simulink model "rx2"  (R2022b)
settings: Solver=FixedStepDiscrete  StartTime=0.0  StopTime=3.3E6  FixedStep=1  RelTol=1e-3  EnableMultiTasking=on
model workspace (MAT data in the model file):
  mwTaskManagerKernelLatency = 0
undefined symbols (not defined in the file or in its folder): Add, jsin, magnitude, rom_pilot_conj_tt, Shift
libraries: hdlsllib x3231, whdlutilities x525, simulink x260, whdlmod x112, whdledac x26, dsphdlmathfun2 x24, commchan3 x1
(part 59 of 59)

== system rx2/process8/decoder/p-p/Subsystem2/Subsystem1/Subsystem1/Subsystem/Subsystem1/Subsystem1 ==
  data : Inport  OutDataTypeStr=data_type
  wr_addr : Inport  Port=2
  wr_en : Inport  Port=3
  rd_addr : Inport  Port=4
  Demux : Demux  Outputs=2
  Mux : Mux  Inputs=2
  Simple Dual Port RAM : hdlsllib/HDL RAMs/Simple Dual Port RAM  ram_size=address_len
  Simple Dual Port RAM1 : hdlsllib/HDL RAMs/Simple Dual Port RAM  ram_size=address_len
  rd_dout : Outport  PortDimensions=2  VectorParamsAs1DForOutWhenUnconnected=off
  wires:
  Mux/1 -> rd_dout/1
  Simple Dual Port RAM/1 -> Mux/1
  Simple Dual Port RAM1/1 -> Mux/2
  data/1 -> Demux/1
  Demux/1 -> Simple Dual Port RAM/1
  Demux/2 -> Simple Dual Port RAM1/1
  wr_addr/1 -> Simple Dual Port RAM1/2, Simple Dual Port RAM/2
  wr_en/1 -> Simple Dual Port RAM/3, Simple Dual Port RAM1/3
  rd_addr/1 -> Simple Dual Port RAM/4, Simple Dual Port RAM1/4

== system rx2/process8/decoder/p-p/Subsystem2/Subsystem1/Subsystem1/Subsystem/Subsystem4/Subsystem ==
  data : Inport  OutDataTypeStr=data_type
  wr_addr : Inport  Port=2
  wr_en : Inport  Port=3
  rd_addr : Inport  Port=4
  Demux : Demux  Outputs=2
  Mux : Mux  Inputs=2
  Simple Dual Port RAM : hdlsllib/HDL RAMs/Simple Dual Port RAM  ram_size=address_len
  Simple Dual Port RAM1 : hdlsllib/HDL RAMs/Simple Dual Port RAM  ram_size=address_len
  rd_dout : Outport  PortDimensions=2  VectorParamsAs1DForOutWhenUnconnected=off
  wires:
  Mux/1 -> rd_dout/1
  Simple Dual Port RAM/1 -> Mux/1
  Simple Dual Port RAM1/1 -> Mux/2
  data/1 -> Demux/1
  Demux/1 -> Simple Dual Port RAM/1
  Demux/2 -> Simple Dual Port RAM1/1
  wr_addr/1 -> Simple Dual Port RAM1/2, Simple Dual Port RAM/2
  wr_en/1 -> Simple Dual Port RAM/3, Simple Dual Port RAM1/3
  rd_addr/1 -> Simple Dual Port RAM/4, Simple Dual Port RAM1/4

== system rx2/process8/decoder/p-p/Subsystem2/Subsystem1/Subsystem1/Subsystem/Subsystem4/Subsystem1 ==
  data : Inport  OutDataTypeStr=data_type
  wr_addr : Inport  Port=2
  wr_en : Inport  Port=3
  rd_addr : Inport  Port=4
  Demux : Demux  Outputs=2
  Mux : Mux  Inputs=2
  Simple Dual Port RAM : hdlsllib/HDL RAMs/Simple Dual Port RAM  ram_size=address_len
  Simple Dual Port RAM1 : hdlsllib/HDL RAMs/Simple Dual Port RAM  ram_size=address_len
  rd_dout : Outport  PortDimensions=2  VectorParamsAs1DForOutWhenUnconnected=off
  wires:
  rd_addr/1 -> Simple Dual Port RAM1/4, Simple Dual Port RAM/4
  wr_en/1 -> Simple Dual Port RAM1/3, Simple Dual Port RAM/3
  wr_addr/1 -> Simple Dual Port RAM/2, Simple Dual Port RAM1/2
  Demux/2 -> Simple Dual Port RAM1/1
  Demux/1 -> Simple Dual Port RAM/1
  data/1 -> Demux/1
  Simple Dual Port RAM1/1 -> Mux/2
  Simple Dual Port RAM/1 -> Mux/1
  Mux/1 -> rd_dout/1

== system rx2/process8/decoder/p-p/Subsystem2/Subsystem1/Subsystem1/Subsystem1/Subsystem1/Subsystem ==
  data : Inport  OutDataTypeStr=data_type
  wr_addr : Inport  Port=2
  wr_en : Inport  Port=3
  rd_addr : Inport  Port=4
  Demux : Demux  Outputs=2
  Mux : Mux  Inputs=2
  Simple Dual Port RAM : hdlsllib/HDL RAMs/Simple Dual Port RAM  ram_size=address_len
  Simple Dual Port RAM1 : hdlsllib/HDL RAMs/Simple Dual Port RAM  ram_size=address_len
  rd_dout : Outport  PortDimensions=2  VectorParamsAs1DForOutWhenUnconnected=off
  wires:
  rd_addr/1 -> Simple Dual Port RAM1/4, Simple Dual Port RAM/4
  wr_en/1 -> Simple Dual Port RAM1/3, Simple Dual Port RAM/3
  wr_addr/1 -> Simple Dual Port RAM/2, Simple Dual Port RAM1/2
  Demux/2 -> Simple Dual Port RAM1/1
  Demux/1 -> Simple Dual Port RAM/1
  data/1 -> Demux/1
  Simple Dual Port RAM1/1 -> Mux/2
  Simple Dual Port RAM/1 -> Mux/1
  Mux/1 -> rd_dout/1

== system rx2/process8/decoder/p-p/Subsystem2/Subsystem1/Subsystem1/Subsystem1/Subsystem1/Subsystem1 ==
  data : Inport  OutDataTypeStr=data_type
  wr_addr : Inport  Port=2
  wr_en : Inport  Port=3
  rd_addr : Inport  Port=4
  Demux : Demux  Outputs=2
  Mux : Mux  Inputs=2
  Simple Dual Port RAM : hdlsllib/HDL RAMs/Simple Dual Port RAM  ram_size=address_len
  Simple Dual Port RAM1 : hdlsllib/HDL RAMs/Simple Dual Port RAM  ram_size=address_len
  rd_dout : Outport  PortDimensions=2  VectorParamsAs1DForOutWhenUnconnected=off
  wires:
  Mux/1 -> rd_dout/1
  Simple Dual Port RAM/1 -> Mux/1
  Simple Dual Port RAM1/1 -> Mux/2
  data/1 -> Demux/1
  Demux/1 -> Simple Dual Port RAM/1
  Demux/2 -> Simple Dual Port RAM1/1
  wr_addr/1 -> Simple Dual Port RAM1/2, Simple Dual Port RAM/2
  wr_en/1 -> Simple Dual Port RAM/3, Simple Dual Port RAM1/3
  rd_addr/1 -> Simple Dual Port RAM/4, Simple Dual Port RAM1/4

== system rx2/process8/decoder/p-p/Subsystem2/Subsystem1/Subsystem1/Subsystem1/Subsystem4/Subsystem ==
  data : Inport  OutDataTypeStr=data_type
  wr_addr : Inport  Port=2
  wr_en : Inport  Port=3
  rd_addr : Inport  Port=4
  Demux : Demux  Outputs=2
  Mux : Mux  Inputs=2
  Simple Dual Port RAM : hdlsllib/HDL RAMs/Simple Dual Port RAM  ram_size=address_len
  Simple Dual Port RAM1 : hdlsllib/HDL RAMs/Simple Dual Port RAM  ram_size=address_len
  rd_dout : Outport  PortDimensions=2  VectorParamsAs1DForOutWhenUnconnected=off
  wires:
  rd_addr/1 -> Simple Dual Port RAM1/4, Simple Dual Port RAM/4
  wr_en/1 -> Simple Dual Port RAM1/3, Simple Dual Port RAM/3
  wr_addr/1 -> Simple Dual Port RAM/2, Simple Dual Port RAM1/2
  Demux/2 -> Simple Dual Port RAM1/1
  Demux/1 -> Simple Dual Port RAM/1
  data/1 -> Demux/1
  Simple Dual Port RAM1/1 -> Mux/2
  Simple Dual Port RAM/1 -> Mux/1
  Mux/1 -> rd_dout/1

== system rx2/process8/decoder/p-p/Subsystem2/Subsystem1/Subsystem1/Subsystem1/Subsystem4/Subsystem1 ==
  data : Inport  OutDataTypeStr=data_type
  wr_addr : Inport  Port=2
  wr_en : Inport  Port=3
  rd_addr : Inport  Port=4
  Demux : Demux  Outputs=2
  Mux : Mux  Inputs=2
  Simple Dual Port RAM : hdlsllib/HDL RAMs/Simple Dual Port RAM  ram_size=address_len
  Simple Dual Port RAM1 : hdlsllib/HDL RAMs/Simple Dual Port RAM  ram_size=address_len
  rd_dout : Outport  PortDimensions=2  VectorParamsAs1DForOutWhenUnconnected=off
  wires:
  Mux/1 -> rd_dout/1
  Simple Dual Port RAM/1 -> Mux/1
  Simple Dual Port RAM1/1 -> Mux/2
  data/1 -> Demux/1
  Demux/1 -> Simple Dual Port RAM/1
  Demux/2 -> Simple Dual Port RAM1/1
  wr_addr/1 -> Simple Dual Port RAM1/2, Simple Dual Port RAM/2
  wr_en/1 -> Simple Dual Port RAM/3, Simple Dual Port RAM1/3
  rd_addr/1 -> Simple Dual Port RAM/4, Simple Dual Port RAM1/4

== system rx2/process8/decoder/p-p/Subsystem2/Subsystem1/Subsystem2/Subsystem/Subsystem1/Subsystem ==
  data : Inport  OutDataTypeStr=data_type
  wr_addr : Inport  Port=2
  wr_en : Inport  Port=3
  rd_addr : Inport  Port=4
  Demux : Demux  Outputs=2
  Mux : Mux  Inputs=2
  Simple Dual Port RAM : hdlsllib/HDL RAMs/Simple Dual Port RAM  ram_size=address_len
  Simple Dual Port RAM1 : hdlsllib/HDL RAMs/Simple Dual Port RAM  ram_size=address_len
  rd_dout : Outport  PortDimensions=2  VectorParamsAs1DForOutWhenUnconnected=off
  wires:
  rd_addr/1 -> Simple Dual Port RAM1/4, Simple Dual Port RAM/4
  wr_en/1 -> Simple Dual Port RAM1/3, Simple Dual Port RAM/3
  wr_addr/1 -> Simple Dual Port RAM/2, Simple Dual Port RAM1/2
  Demux/2 -> Simple Dual Port RAM1/1
  Demux/1 -> Simple Dual Port RAM/1
  data/1 -> Demux/1
  Simple Dual Port RAM1/1 -> Mux/2
  Simple Dual Port RAM/1 -> Mux/1
  Mux/1 -> rd_dout/1

== system rx2/process8/decoder/p-p/Subsystem2/Subsystem1/Subsystem2/Subsystem/Subsystem1/Subsystem1 ==
  data : Inport  OutDataTypeStr=data_type
  wr_addr : Inport  Port=2
  wr_en : Inport  Port=3
  rd_addr : Inport  Port=4
  Demux : Demux  Outputs=2
  Mux : Mux  Inputs=2
  Simple Dual Port RAM : hdlsllib/HDL RAMs/Simple Dual Port RAM  ram_size=address_len
  Simple Dual Port RAM1 : hdlsllib/HDL RAMs/Simple Dual Port RAM  ram_size=address_len
  rd_dout : Outport  PortDimensions=2  VectorParamsAs1DForOutWhenUnconnected=off
  wires:
  Mux/1 -> rd_dout/1
  Simple Dual Port RAM/1 -> Mux/1
  Simple Dual Port RAM1/1 -> Mux/2
  data/1 -> Demux/1
  Demux/1 -> Simple Dual Port RAM/1
  Demux/2 -> Simple Dual Port RAM1/1
  wr_addr/1 -> Simple Dual Port RAM1/2, Simple Dual Port RAM/2
  wr_en/1 -> Simple Dual Port RAM/3, Simple Dual Port RAM1/3
  rd_addr/1 -> Simple Dual Port RAM/4, Simple Dual Port RAM1/4

== system rx2/process8/decoder/p-p/Subsystem2/Subsystem1/Subsystem2/Subsystem/Subsystem4/Subsystem ==
  data : Inport  OutDataTypeStr=data_type
  wr_addr : Inport  Port=2
  wr_en : Inport  Port=3
  rd_addr : Inport  Port=4
  Demux : Demux  Outputs=2
  Mux : Mux  Inputs=2
  Simple Dual Port RAM : hdlsllib/HDL RAMs/Simple Dual Port RAM  ram_size=address_len
  Simple Dual Port RAM1 : hdlsllib/HDL RAMs/Simple Dual Port RAM  ram_size=address_len
  rd_dout : Outport  PortDimensions=2  VectorParamsAs1DForOutWhenUnconnected=off
  wires:
  Mux/1 -> rd_dout/1
  Simple Dual Port RAM/1 -> Mux/1
  Simple Dual Port RAM1/1 -> Mux/2
  data/1 -> Demux/1
  Demux/1 -> Simple Dual Port RAM/1
  Demux/2 -> Simple Dual Port RAM1/1
  wr_addr/1 -> Simple Dual Port RAM1/2, Simple Dual Port RAM/2
  wr_en/1 -> Simple Dual Port RAM/3, Simple Dual Port RAM1/3
  rd_addr/1 -> Simple Dual Port RAM/4, Simple Dual Port RAM1/4

== system rx2/process8/decoder/p-p/Subsystem2/Subsystem1/Subsystem2/Subsystem/Subsystem4/Subsystem1 ==
  data : Inport  OutDataTypeStr=data_type
  wr_addr : Inport  Port=2
  wr_en : Inport  Port=3
  rd_addr : Inport  Port=4
  Demux : Demux  Outputs=2
  Mux : Mux  Inputs=2
  Simple Dual Port RAM : hdlsllib/HDL RAMs/Simple Dual Port RAM  ram_size=address_len
  Simple Dual Port RAM1 : hdlsllib/HDL RAMs/Simple Dual Port RAM  ram_size=address_len
  rd_dout : Outport  PortDimensions=2  VectorParamsAs1DForOutWhenUnconnected=off
  wires:
  rd_addr/1 -> Simple Dual Port RAM1/4, Simple Dual Port RAM/4
  wr_en/1 -> Simple Dual Port RAM1/3, Simple Dual Port RAM/3
  wr_addr/1 -> Simple Dual Port RAM/2, Simple Dual Port RAM1/2
  Demux/2 -> Simple Dual Port RAM1/1
  Demux/1 -> Simple Dual Port RAM/1
  data/1 -> Demux/1
  Simple Dual Port RAM1/1 -> Mux/2
  Simple Dual Port RAM/1 -> Mux/1
  Mux/1 -> rd_dout/1

== system rx2/process8/decoder/p-p/Subsystem2/Subsystem1/Subsystem2/Subsystem1/Subsystem1/Subsystem ==
  data : Inport  OutDataTypeStr=data_type
  wr_addr : Inport  Port=2
  wr_en : Inport  Port=3
  rd_addr : Inport  Port=4
  Demux : Demux  Outputs=2
  Mux : Mux  Inputs=2
  Simple Dual Port RAM : hdlsllib/HDL RAMs/Simple Dual Port RAM  ram_size=address_len
  Simple Dual Port RAM1 : hdlsllib/HDL RAMs/Simple Dual Port RAM  ram_size=address_len
  rd_dout : Outport  PortDimensions=2  VectorParamsAs1DForOutWhenUnconnected=off
  wires:
  rd_addr/1 -> Simple Dual Port RAM1/4, Simple Dual Port RAM/4
  wr_en/1 -> Simple Dual Port RAM1/3, Simple Dual Port RAM/3
  wr_addr/1 -> Simple Dual Port RAM/2, Simple Dual Port RAM1/2
  Demux/2 -> Simple Dual Port RAM1/1
  Demux/1 -> Simple Dual Port RAM/1
  data/1 -> Demux/1
  Simple Dual Port RAM1/1 -> Mux/2
  Simple Dual Port RAM/1 -> Mux/1
  Mux/1 -> rd_dout/1

== system rx2/process8/decoder/p-p/Subsystem2/Subsystem1/Subsystem2/Subsystem1/Subsystem1/Subsystem1 ==
  data : Inport  OutDataTypeStr=data_type
  wr_addr : Inport  Port=2
  wr_en : Inport  Port=3
  rd_addr : Inport  Port=4
  Demux : Demux  Outputs=2
  Mux : Mux  Inputs=2
  Simple Dual Port RAM : hdlsllib/HDL RAMs/Simple Dual Port RAM  ram_size=address_len
  Simple Dual Port RAM1 : hdlsllib/HDL RAMs/Simple Dual Port RAM  ram_size=address_len
  rd_dout : Outport  PortDimensions=2  VectorParamsAs1DForOutWhenUnconnected=off
  wires:
  Mux/1 -> rd_dout/1
  Simple Dual Port RAM/1 -> Mux/1
  Simple Dual Port RAM1/1 -> Mux/2
  data/1 -> Demux/1
  Demux/1 -> Simple Dual Port RAM/1
  Demux/2 -> Simple Dual Port RAM1/1
  wr_addr/1 -> Simple Dual Port RAM1/2, Simple Dual Port RAM/2
  wr_en/1 -> Simple Dual Port RAM/3, Simple Dual Port RAM1/3
  rd_addr/1 -> Simple Dual Port RAM/4, Simple Dual Port RAM1/4

== system rx2/process8/decoder/p-p/Subsystem2/Subsystem1/Subsystem2/Subsystem1/Subsystem4/Subsystem ==
  data : Inport  OutDataTypeStr=data_type
  wr_addr : Inport  Port=2
  wr_en : Inport  Port=3
  rd_addr : Inport  Port=4
  Demux : Demux  Outputs=2
  Mux : Mux  Inputs=2
  Simple Dual Port RAM : hdlsllib/HDL RAMs/Simple Dual Port RAM  ram_size=address_len
  Simple Dual Port RAM1 : hdlsllib/HDL RAMs/Simple Dual Port RAM  ram_size=address_len
  rd_dout : Outport  PortDimensions=2  VectorParamsAs1DForOutWhenUnconnected=off
  wires:
  rd_addr/1 -> Simple Dual Port RAM1/4, Simple Dual Port RAM/4
  wr_en/1 -> Simple Dual Port RAM1/3, Simple Dual Port RAM/3
  wr_addr/1 -> Simple Dual Port RAM/2, Simple Dual Port RAM1/2
  Demux/2 -> Simple Dual Port RAM1/1
  Demux/1 -> Simple Dual Port RAM/1
  data/1 -> Demux/1
  Simple Dual Port RAM1/1 -> Mux/2
  Simple Dual Port RAM/1 -> Mux/1
  Mux/1 -> rd_dout/1

== system rx2/process8/decoder/p-p/Subsystem2/Subsystem1/Subsystem2/Subsystem1/Subsystem4/Subsystem1 ==
  data : Inport  OutDataTypeStr=data_type
  wr_addr : Inport  Port=2
  wr_en : Inport  Port=3
  rd_addr : Inport  Port=4
  Demux : Demux  Outputs=2
  Mux : Mux  Inputs=2
  Simple Dual Port RAM : hdlsllib/HDL RAMs/Simple Dual Port RAM  ram_size=address_len
  Simple Dual Port RAM1 : hdlsllib/HDL RAMs/Simple Dual Port RAM  ram_size=address_len
  rd_dout : Outport  PortDimensions=2  VectorParamsAs1DForOutWhenUnconnected=off
  wires:
  Mux/1 -> rd_dout/1
  Simple Dual Port RAM/1 -> Mux/1
  Simple Dual Port RAM1/1 -> Mux/2
  data/1 -> Demux/1
  Demux/1 -> Simple Dual Port RAM/1
  Demux/2 -> Simple Dual Port RAM1/1
  wr_addr/1 -> Simple Dual Port RAM1/2, Simple Dual Port RAM/2
  wr_en/1 -> Simple Dual Port RAM/3, Simple Dual Port RAM1/3
  rd_addr/1 -> Simple Dual Port RAM/4, Simple Dual Port RAM1/4

== system rx2/process9/decoder/p-p/Subsystem2/Subsystem/Subsystem1/Subsystem/Subsystem1/Subsystem ==
  data : Inport  OutDataTypeStr=data_type
  wr_addr : Inport  Port=2
  wr_en : Inport  Port=3
  rd_addr : Inport  Port=4
  Demux : Demux  Outputs=2
  Mux : Mux  Inputs=2
  Simple Dual Port RAM : hdlsllib/HDL RAMs/Simple Dual Port RAM  ram_size=address_len
  Simple Dual Port RAM1 : hdlsllib/HDL RAMs/Simple Dual Port RAM  ram_size=address_len
  rd_dout : Outport  PortDimensions=2  VectorParamsAs1DForOutWhenUnconnected=off
  wires:
  Mux/1 -> rd_dout/1
  Simple Dual Port RAM/1 -> Mux/1
  Simple Dual Port RAM1/1 -> Mux/2
  data/1 -> Demux/1
  Demux/1 -> Simple Dual Port RAM/1
  Demux/2 -> Simple Dual Port RAM1/1
  wr_addr/1 -> Simple Dual Port RAM1/2, Simple Dual Port RAM/2
  wr_en/1 -> Simple Dual Port RAM/3, Simple Dual Port RAM1/3
  rd_addr/1 -> Simple Dual Port RAM/4, Simple Dual Port RAM1/4

== system rx2/process9/decoder/p-p/Subsystem2/Subsystem/Subsystem1/Subsystem/Subsystem1/Subsystem1 ==
  data : Inport  OutDataTypeStr=data_type
  wr_addr : Inport  Port=2
  wr_en : Inport  Port=3
  rd_addr : Inport  Port=4
  Demux : Demux  Outputs=2
  Mux : Mux  Inputs=2
  Simple Dual Port RAM : hdlsllib/HDL RAMs/Simple Dual Port RAM  ram_size=address_len
  Simple Dual Port RAM1 : hdlsllib/HDL RAMs/Simple Dual Port RAM  ram_size=address_len
  rd_dout : Outport  PortDimensions=2  VectorParamsAs1DForOutWhenUnconnected=off
  wires:
  rd_addr/1 -> Simple Dual Port RAM1/4, Simple Dual Port RAM/4
  wr_en/1 -> Simple Dual Port RAM1/3, Simple Dual Port RAM/3
  wr_addr/1 -> Simple Dual Port RAM/2, Simple Dual Port RAM1/2
  Demux/2 -> Simple Dual Port RAM1/1
  Demux/1 -> Simple Dual Port RAM/1
  data/1 -> Demux/1
  Simple Dual Port RAM1/1 -> Mux/2
  Simple Dual Port RAM/1 -> Mux/1
  Mux/1 -> rd_dout/1

== system rx2/process9/decoder/p-p/Subsystem2/Subsystem/Subsystem1/Subsystem/Subsystem4/Subsystem ==
  data : Inport  OutDataTypeStr=data_type
  wr_addr : Inport  Port=2
  wr_en : Inport  Port=3
  rd_addr : Inport  Port=4
  Demux : Demux  Outputs=2
  Mux : Mux  Inputs=2
  Simple Dual Port RAM : hdlsllib/HDL RAMs/Simple Dual Port RAM  ram_size=address_len
  Simple Dual Port RAM1 : hdlsllib/HDL RAMs/Simple Dual Port RAM  ram_size=address_len
  rd_dout : Outport  PortDimensions=2  VectorParamsAs1DForOutWhenUnconnected=off
  wires:
  rd_addr/1 -> Simple Dual Port RAM1/4, Simple Dual Port RAM/4
  wr_en/1 -> Simple Dual Port RAM1/3, Simple Dual Port RAM/3
  wr_addr/1 -> Simple Dual Port RAM/2, Simple Dual Port RAM1/2
  Demux/2 -> Simple Dual Port RAM1/1
  Demux/1 -> Simple Dual Port RAM/1
  data/1 -> Demux/1
  Simple Dual Port RAM1/1 -> Mux/2
  Simple Dual Port RAM/1 -> Mux/1
  Mux/1 -> rd_dout/1

== system rx2/process9/decoder/p-p/Subsystem2/Subsystem/Subsystem1/Subsystem/Subsystem4/Subsystem1 ==
  data : Inport  OutDataTypeStr=data_type
  wr_addr : Inport  Port=2
  wr_en : Inport  Port=3
  rd_addr : Inport  Port=4
  Demux : Demux  Outputs=2
  Mux : Mux  Inputs=2
  Simple Dual Port RAM : hdlsllib/HDL RAMs/Simple Dual Port RAM  ram_size=address_len
  Simple Dual Port RAM1 : hdlsllib/HDL RAMs/Simple Dual Port RAM  ram_size=address_len
  rd_dout : Outport  PortDimensions=2  VectorParamsAs1DForOutWhenUnconnected=off
  wires:
  Mux/1 -> rd_dout/1
  Simple Dual Port RAM/1 -> Mux/1
  Simple Dual Port RAM1/1 -> Mux/2
  data/1 -> Demux/1
  Demux/1 -> Simple Dual Port RAM/1
  Demux/2 -> Simple Dual Port RAM1/1
  wr_addr/1 -> Simple Dual Port RAM1/2, Simple Dual Port RAM/2
  wr_en/1 -> Simple Dual Port RAM/3, Simple Dual Port RAM1/3
  rd_addr/1 -> Simple Dual Port RAM/4, Simple Dual Port RAM1/4

== system rx2/process9/decoder/p-p/Subsystem2/Subsystem/Subsystem1/Subsystem1/Subsystem1/Subsystem ==
  data : Inport  OutDataTypeStr=data_type
  wr_addr : Inport  Port=2
  wr_en : Inport  Port=3
  rd_addr : Inport  Port=4
  Demux : Demux  Outputs=2
  Mux : Mux  Inputs=2
  Simple Dual Port RAM : hdlsllib/HDL RAMs/Simple Dual Port RAM  ram_size=address_len
  Simple Dual Port RAM1 : hdlsllib/HDL RAMs/Simple Dual Port RAM  ram_size=address_len
  rd_dout : Outport  PortDimensions=2  VectorParamsAs1DForOutWhenUnconnected=off
  wires:
  Mux/1 -> rd_dout/1
  Simple Dual Port RAM/1 -> Mux/1
  Simple Dual Port RAM1/1 -> Mux/2
  data/1 -> Demux/1
  Demux/1 -> Simple Dual Port RAM/1
  Demux/2 -> Simple Dual Port RAM1/1
  wr_addr/1 -> Simple Dual Port RAM1/2, Simple Dual Port RAM/2
  wr_en/1 -> Simple Dual Port RAM/3, Simple Dual Port RAM1/3
  rd_addr/1 -> Simple Dual Port RAM/4, Simple Dual Port RAM1/4

== system rx2/process9/decoder/p-p/Subsystem2/Subsystem/Subsystem1/Subsystem1/Subsystem1/Subsystem1 ==
  data : Inport  OutDataTypeStr=data_type
  wr_addr : Inport  Port=2
  wr_en : Inport  Port=3
  rd_addr : Inport  Port=4
  Demux : Demux  Outputs=2
  Mux : Mux  Inputs=2
  Simple Dual Port RAM : hdlsllib/HDL RAMs/Simple Dual Port RAM  ram_size=address_len
  Simple Dual Port RAM1 : hdlsllib/HDL RAMs/Simple Dual Port RAM  ram_size=address_len
  rd_dout : Outport  PortDimensions=2  VectorParamsAs1DForOutWhenUnconnected=off
  wires:
  rd_addr/1 -> Simple Dual Port RAM1/4, Simple Dual Port RAM/4
  wr_en/1 -> Simple Dual Port RAM1/3, Simple Dual Port RAM/3
  wr_addr/1 -> Simple Dual Port RAM/2, Simple Dual Port RAM1/2
  Demux/2 -> Simple Dual Port RAM1/1
  Demux/1 -> Simple Dual Port RAM/1
  data/1 -> Demux/1
  Simple Dual Port RAM1/1 -> Mux/2
  Simple Dual Port RAM/1 -> Mux/1
  Mux/1 -> rd_dout/1

== system rx2/process9/decoder/p-p/Subsystem2/Subsystem/Subsystem1/Subsystem1/Subsystem4/Subsystem ==
  data : Inport  OutDataTypeStr=data_type
  wr_addr : Inport  Port=2
  wr_en : Inport  Port=3
  rd_addr : Inport  Port=4
  Demux : Demux  Outputs=2
  Mux : Mux  Inputs=2
  Simple Dual Port RAM : hdlsllib/HDL RAMs/Simple Dual Port RAM  ram_size=address_len
  Simple Dual Port RAM1 : hdlsllib/HDL RAMs/Simple Dual Port RAM  ram_size=address_len
  rd_dout : Outport  PortDimensions=2  VectorParamsAs1DForOutWhenUnconnected=off
  wires:
  Mux/1 -> rd_dout/1
  Simple Dual Port RAM/1 -> Mux/1
  Simple Dual Port RAM1/1 -> Mux/2
  data/1 -> Demux/1
  Demux/1 -> Simple Dual Port RAM/1
  Demux/2 -> Simple Dual Port RAM1/1
  wr_addr/1 -> Simple Dual Port RAM1/2, Simple Dual Port RAM/2
  wr_en/1 -> Simple Dual Port RAM/3, Simple Dual Port RAM1/3
  rd_addr/1 -> Simple Dual Port RAM/4, Simple Dual Port RAM1/4

== system rx2/process9/decoder/p-p/Subsystem2/Subsystem/Subsystem1/Subsystem1/Subsystem4/Subsystem1 ==
  data : Inport  OutDataTypeStr=data_type
  wr_addr : Inport  Port=2
  wr_en : Inport  Port=3
  rd_addr : Inport  Port=4
  Demux : Demux  Outputs=2
  Mux : Mux  Inputs=2
  Simple Dual Port RAM : hdlsllib/HDL RAMs/Simple Dual Port RAM  ram_size=address_len
  Simple Dual Port RAM1 : hdlsllib/HDL RAMs/Simple Dual Port RAM  ram_size=address_len
  rd_dout : Outport  PortDimensions=2  VectorParamsAs1DForOutWhenUnconnected=off
  wires:
  rd_addr/1 -> Simple Dual Port RAM1/4, Simple Dual Port RAM/4
  wr_en/1 -> Simple Dual Port RAM1/3, Simple Dual Port RAM/3
  wr_addr/1 -> Simple Dual Port RAM/2, Simple Dual Port RAM1/2
  Demux/2 -> Simple Dual Port RAM1/1
  Demux/1 -> Simple Dual Port RAM/1
  data/1 -> Demux/1
  Simple Dual Port RAM1/1 -> Mux/2
  Simple Dual Port RAM/1 -> Mux/1
  Mux/1 -> rd_dout/1

== system rx2/process9/decoder/p-p/Subsystem2/Subsystem/Subsystem2/Subsystem/Subsystem1/Subsystem ==
  data : Inport  OutDataTypeStr=data_type
  wr_addr : Inport  Port=2
  wr_en : Inport  Port=3
  rd_addr : Inport  Port=4
  Demux : Demux  Outputs=2
  Mux : Mux  Inputs=2
  Simple Dual Port RAM : hdlsllib/HDL RAMs/Simple Dual Port RAM  ram_size=address_len
  Simple Dual Port RAM1 : hdlsllib/HDL RAMs/Simple Dual Port RAM  ram_size=address_len
  rd_dout : Outport  PortDimensions=2  VectorParamsAs1DForOutWhenUnconnected=off
  wires:
  Mux/1 -> rd_dout/1
  Simple Dual Port RAM/1 -> Mux/1
  Simple Dual Port RAM1/1 -> Mux/2
  data/1 -> Demux/1
  Demux/1 -> Simple Dual Port RAM/1
  Demux/2 -> Simple Dual Port RAM1/1
  wr_addr/1 -> Simple Dual Port RAM1/2, Simple Dual Port RAM/2
  wr_en/1 -> Simple Dual Port RAM/3, Simple Dual Port RAM1/3
  rd_addr/1 -> Simple Dual Port RAM/4, Simple Dual Port RAM1/4

== system rx2/process9/decoder/p-p/Subsystem2/Subsystem/Subsystem2/Subsystem/Subsystem1/Subsystem1 ==
  data : Inport  OutDataTypeStr=data_type
  wr_addr : Inport  Port=2
  wr_en : Inport  Port=3
  rd_addr : Inport  Port=4
  Demux : Demux  Outputs=2
  Mux : Mux  Inputs=2
  Simple Dual Port RAM : hdlsllib/HDL RAMs/Simple Dual Port RAM  ram_size=address_len
  Simple Dual Port RAM1 : hdlsllib/HDL RAMs/Simple Dual Port RAM  ram_size=address_len
  rd_dout : Outport  PortDimensions=2  VectorParamsAs1DForOutWhenUnconnected=off
  wires:
  rd_addr/1 -> Simple Dual Port RAM1/4, Simple Dual Port RAM/4
  wr_en/1 -> Simple Dual Port RAM1/3, Simple Dual Port RAM/3
  wr_addr/1 -> Simple Dual Port RAM/2, Simple Dual Port RAM1/2
  Demux/2 -> Simple Dual Port RAM1/1
  Demux/1 -> Simple Dual Port RAM/1
  data/1 -> Demux/1
  Simple Dual Port RAM1/1 -> Mux/2
  Simple Dual Port RAM/1 -> Mux/1
  Mux/1 -> rd_dout/1

== system rx2/process9/decoder/p-p/Subsystem2/Subsystem/Subsystem2/Subsystem/Subsystem4/Subsystem ==
  data : Inport  OutDataTypeStr=data_type
  wr_addr : Inport  Port=2
  wr_en : Inport  Port=3
  rd_addr : Inport  Port=4
  Demux : Demux  Outputs=2
  Mux : Mux  Inputs=2
  Simple Dual Port RAM : hdlsllib/HDL RAMs/Simple Dual Port RAM  ram_size=address_len
  Simple Dual Port RAM1 : hdlsllib/HDL RAMs/Simple Dual Port RAM  ram_size=address_len
  rd_dout : Outport  PortDimensions=2  VectorParamsAs1DForOutWhenUnconnected=off
  wires:
  rd_addr/1 -> Simple Dual Port RAM1/4, Simple Dual Port RAM/4
  wr_en/1 -> Simple Dual Port RAM1/3, Simple Dual Port RAM/3
  wr_addr/1 -> Simple Dual Port RAM/2, Simple Dual Port RAM1/2
  Demux/2 -> Simple Dual Port RAM1/1
  Demux/1 -> Simple Dual Port RAM/1
  data/1 -> Demux/1
  Simple Dual Port RAM1/1 -> Mux/2
  Simple Dual Port RAM/1 -> Mux/1
  Mux/1 -> rd_dout/1

== system rx2/process9/decoder/p-p/Subsystem2/Subsystem/Subsystem2/Subsystem/Subsystem4/Subsystem1 ==
  data : Inport  OutDataTypeStr=data_type
  wr_addr : Inport  Port=2
  wr_en : Inport  Port=3
  rd_addr : Inport  Port=4
  Demux : Demux  Outputs=2
  Mux : Mux  Inputs=2
  Simple Dual Port RAM : hdlsllib/HDL RAMs/Simple Dual Port RAM  ram_size=address_len
  Simple Dual Port RAM1 : hdlsllib/HDL RAMs/Simple Dual Port RAM  ram_size=address_len
  rd_dout : Outport  PortDimensions=2  VectorParamsAs1DForOutWhenUnconnected=off
  wires:
  Mux/1 -> rd_dout/1
  Simple Dual Port RAM/1 -> Mux/1
  Simple Dual Port RAM1/1 -> Mux/2
  data/1 -> Demux/1
  Demux/1 -> Simple Dual Port RAM/1
  Demux/2 -> Simple Dual Port RAM1/1
  wr_addr/1 -> Simple Dual Port RAM1/2, Simple Dual Port RAM/2
  wr_en/1 -> Simple Dual Port RAM/3, Simple Dual Port RAM1/3
  rd_addr/1 -> Simple Dual Port RAM/4, Simple Dual Port RAM1/4

== system rx2/process9/decoder/p-p/Subsystem2/Subsystem/Subsystem2/Subsystem1/Subsystem1/Subsystem ==
  data : Inport  OutDataTypeStr=data_type
  wr_addr : Inport  Port=2
  wr_en : Inport  Port=3
  rd_addr : Inport  Port=4
  Demux : Demux  Outputs=2
  Mux : Mux  Inputs=2
  Simple Dual Port RAM : hdlsllib/HDL RAMs/Simple Dual Port RAM  ram_size=address_len
  Simple Dual Port RAM1 : hdlsllib/HDL RAMs/Simple Dual Port RAM  ram_size=address_len
  rd_dout : Outport  PortDimensions=2  VectorParamsAs1DForOutWhenUnconnected=off
  wires:
  Mux/1 -> rd_dout/1
  Simple Dual Port RAM/1 -> Mux/1
  Simple Dual Port RAM1/1 -> Mux/2
  data/1 -> Demux/1
  Demux/1 -> Simple Dual Port RAM/1
  Demux/2 -> Simple Dual Port RAM1/1
  wr_addr/1 -> Simple Dual Port RAM1/2, Simple Dual Port RAM/2
  wr_en/1 -> Simple Dual Port RAM/3, Simple Dual Port RAM1/3
  rd_addr/1 -> Simple Dual Port RAM/4, Simple Dual Port RAM1/4

== system rx2/process9/decoder/p-p/Subsystem2/Subsystem/Subsystem2/Subsystem1/Subsystem1/Subsystem1 ==
  data : Inport  OutDataTypeStr=data_type
  wr_addr : Inport  Port=2
  wr_en : Inport  Port=3
  rd_addr : Inport  Port=4
  Demux : Demux  Outputs=2
  Mux : Mux  Inputs=2
  Simple Dual Port RAM : hdlsllib/HDL RAMs/Simple Dual Port RAM  ram_size=address_len
  Simple Dual Port RAM1 : hdlsllib/HDL RAMs/Simple Dual Port RAM  ram_size=address_len
  rd_dout : Outport  PortDimensions=2  VectorParamsAs1DForOutWhenUnconnected=off
  wires:
  rd_addr/1 -> Simple Dual Port RAM1/4, Simple Dual Port RAM/4
  wr_en/1 -> Simple Dual Port RAM1/3, Simple Dual Port RAM/3
  wr_addr/1 -> Simple Dual Port RAM/2, Simple Dual Port RAM1/2
  Demux/2 -> Simple Dual Port RAM1/1
  Demux/1 -> Simple Dual Port RAM/1
  data/1 -> Demux/1
  Simple Dual Port RAM1/1 -> Mux/2
  Simple Dual Port RAM/1 -> Mux/1
  Mux/1 -> rd_dout/1

== system rx2/process9/decoder/p-p/Subsystem2/Subsystem/Subsystem2/Subsystem1/Subsystem4/Subsystem ==
  data : Inport  OutDataTypeStr=data_type
  wr_addr : Inport  Port=2
  wr_en : Inport  Port=3
  rd_addr : Inport  Port=4
  Demux : Demux  Outputs=2
  Mux : Mux  Inputs=2
  Simple Dual Port RAM : hdlsllib/HDL RAMs/Simple Dual Port RAM  ram_size=address_len
  Simple Dual Port RAM1 : hdlsllib/HDL RAMs/Simple Dual Port RAM  ram_size=address_len
  rd_dout : Outport  PortDimensions=2  VectorParamsAs1DForOutWhenUnconnected=off
  wires:
  Mux/1 -> rd_dout/1
  Simple Dual Port RAM/1 -> Mux/1
  Simple Dual Port RAM1/1 -> Mux/2
  data/1 -> Demux/1
  Demux/1 -> Simple Dual Port RAM/1
  Demux/2 -> Simple Dual Port RAM1/1
  wr_addr/1 -> Simple Dual Port RAM1/2, Simple Dual Port RAM/2
  wr_en/1 -> Simple Dual Port RAM/3, Simple Dual Port RAM1/3
  rd_addr/1 -> Simple Dual Port RAM/4, Simple Dual Port RAM1/4

== system rx2/process9/decoder/p-p/Subsystem2/Subsystem/Subsystem2/Subsystem1/Subsystem4/Subsystem1 ==
  data : Inport  OutDataTypeStr=data_type
  wr_addr : Inport  Port=2
  wr_en : Inport  Port=3
  rd_addr : Inport  Port=4
  Demux : Demux  Outputs=2
  Mux : Mux  Inputs=2
  Simple Dual Port RAM : hdlsllib/HDL RAMs/Simple Dual Port RAM  ram_size=address_len
  Simple Dual Port RAM1 : hdlsllib/HDL RAMs/Simple Dual Port RAM  ram_size=address_len
  rd_dout : Outport  PortDimensions=2  VectorParamsAs1DForOutWhenUnconnected=off
  wires:
  rd_addr/1 -> Simple Dual Port RAM1/4, Simple Dual Port RAM/4
  wr_en/1 -> Simple Dual Port RAM1/3, Simple Dual Port RAM/3
  wr_addr/1 -> Simple Dual Port RAM/2, Simple Dual Port RAM1/2
  Demux/2 -> Simple Dual Port RAM1/1
  Demux/1 -> Simple Dual Port RAM/1
  data/1 -> Demux/1
  Simple Dual Port RAM1/1 -> Mux/2
  Simple Dual Port RAM/1 -> Mux/1
  Mux/1 -> rd_dout/1

== system rx2/process9/decoder/p-p/Subsystem2/Subsystem1/Subsystem1/Subsystem/Subsystem1/Subsystem ==
  data : Inport  OutDataTypeStr=data_type
  wr_addr : Inport  Port=2
  wr_en : Inport  Port=3
  rd_addr : Inport  Port=4
  Demux : Demux  Outputs=2
  Mux : Mux  Inputs=2
  Simple Dual Port RAM : hdlsllib/HDL RAMs/Simple Dual Port RAM  ram_size=address_len
  Simple Dual Port RAM1 : hdlsllib/HDL RAMs/Simple Dual Port RAM  ram_size=address_len
  rd_dout : Outport  PortDimensions=2  VectorParamsAs1DForOutWhenUnconnected=off
  wires:
  Mux/1 -> rd_dout/1
  Simple Dual Port RAM/1 -> Mux/1
  Simple Dual Port RAM1/1 -> Mux/2
  data/1 -> Demux/1
  Demux/1 -> Simple Dual Port RAM/1
  Demux/2 -> Simple Dual Port RAM1/1
  wr_addr/1 -> Simple Dual Port RAM1/2, Simple Dual Port RAM/2
  wr_en/1 -> Simple Dual Port RAM/3, Simple Dual Port RAM1/3
  rd_addr/1 -> Simple Dual Port RAM/4, Simple Dual Port RAM1/4

== system rx2/process9/decoder/p-p/Subsystem2/Subsystem1/Subsystem1/Subsystem/Subsystem1/Subsystem1 ==
  data : Inport  OutDataTypeStr=data_type
  wr_addr : Inport  Port=2
  wr_en : Inport  Port=3
  rd_addr : Inport  Port=4
  Demux : Demux  Outputs=2
  Mux : Mux  Inputs=2
  Simple Dual Port RAM : hdlsllib/HDL RAMs/Simple Dual Port RAM  ram_size=address_len
  Simple Dual Port RAM1 : hdlsllib/HDL RAMs/Simple Dual Port RAM  ram_size=address_len
  rd_dout : Outport  PortDimensions=2  VectorParamsAs1DForOutWhenUnconnected=off
  wires:
  rd_addr/1 -> Simple Dual Port RAM1/4, Simple Dual Port RAM/4
  wr_en/1 -> Simple Dual Port RAM1/3, Simple Dual Port RAM/3
  wr_addr/1 -> Simple Dual Port RAM/2, Simple Dual Port RAM1/2
  Demux/2 -> Simple Dual Port RAM1/1
  Demux/1 -> Simple Dual Port RAM/1
  data/1 -> Demux/1
  Simple Dual Port RAM1/1 -> Mux/2
  Simple Dual Port RAM/1 -> Mux/1
  Mux/1 -> rd_dout/1

== system rx2/process9/decoder/p-p/Subsystem2/Subsystem1/Subsystem1/Subsystem/Subsystem4/Subsystem ==
  data : Inport  OutDataTypeStr=data_type
  wr_addr : Inport  Port=2
  wr_en : Inport  Port=3
  rd_addr : Inport  Port=4
  Demux : Demux  Outputs=2
  Mux : Mux  Inputs=2
  Simple Dual Port RAM : hdlsllib/HDL RAMs/Simple Dual Port RAM  ram_size=address_len
  Simple Dual Port RAM1 : hdlsllib/HDL RAMs/Simple Dual Port RAM  ram_size=address_len
  rd_dout : Outport  PortDimensions=2  VectorParamsAs1DForOutWhenUnconnected=off
  wires:
  rd_addr/1 -> Simple Dual Port RAM1/4, Simple Dual Port RAM/4
  wr_en/1 -> Simple Dual Port RAM1/3, Simple Dual Port RAM/3
  wr_addr/1 -> Simple Dual Port RAM/2, Simple Dual Port RAM1/2
  Demux/2 -> Simple Dual Port RAM1/1
  Demux/1 -> Simple Dual Port RAM/1
  data/1 -> Demux/1
  Simple Dual Port RAM1/1 -> Mux/2
  Simple Dual Port RAM/1 -> Mux/1
  Mux/1 -> rd_dout/1

== system rx2/process9/decoder/p-p/Subsystem2/Subsystem1/Subsystem1/Subsystem/Subsystem4/Subsystem1 ==
  data : Inport  OutDataTypeStr=data_type
  wr_addr : Inport  Port=2
  wr_en : Inport  Port=3
  rd_addr : Inport  Port=4
  Demux : Demux  Outputs=2
  Mux : Mux  Inputs=2
  Simple Dual Port RAM : hdlsllib/HDL RAMs/Simple Dual Port RAM  ram_size=address_len
  Simple Dual Port RAM1 : hdlsllib/HDL RAMs/Simple Dual Port RAM  ram_size=address_len
  rd_dout : Outport  PortDimensions=2  VectorParamsAs1DForOutWhenUnconnected=off
  wires:
  Mux/1 -> rd_dout/1
  Simple Dual Port RAM/1 -> Mux/1
  Simple Dual Port RAM1/1 -> Mux/2
  data/1 -> Demux/1
  Demux/1 -> Simple Dual Port RAM/1
  Demux/2 -> Simple Dual Port RAM1/1
  wr_addr/1 -> Simple Dual Port RAM1/2, Simple Dual Port RAM/2
  wr_en/1 -> Simple Dual Port RAM/3, Simple Dual Port RAM1/3
  rd_addr/1 -> Simple Dual Port RAM/4, Simple Dual Port RAM1/4

== system rx2/process9/decoder/p-p/Subsystem2/Subsystem1/Subsystem1/Subsystem1/Subsystem1/Subsystem ==
  data : Inport  OutDataTypeStr=data_type
  wr_addr : Inport  Port=2
  wr_en : Inport  Port=3
  rd_addr : Inport  Port=4
  Demux : Demux  Outputs=2
  Mux : Mux  Inputs=2
  Simple Dual Port RAM : hdlsllib/HDL RAMs/Simple Dual Port RAM  ram_size=address_len
  Simple Dual Port RAM1 : hdlsllib/HDL RAMs/Simple Dual Port RAM  ram_size=address_len
  rd_dout : Outport  PortDimensions=2  VectorParamsAs1DForOutWhenUnconnected=off
  wires:
  Mux/1 -> rd_dout/1
  Simple Dual Port RAM/1 -> Mux/1
  Simple Dual Port RAM1/1 -> Mux/2
  data/1 -> Demux/1
  Demux/1 -> Simple Dual Port RAM/1
  Demux/2 -> Simple Dual Port RAM1/1
  wr_addr/1 -> Simple Dual Port RAM1/2, Simple Dual Port RAM/2
  wr_en/1 -> Simple Dual Port RAM/3, Simple Dual Port RAM1/3
  rd_addr/1 -> Simple Dual Port RAM/4, Simple Dual Port RAM1/4

== system rx2/process9/decoder/p-p/Subsystem2/Subsystem1/Subsystem1/Subsystem1/Subsystem1/Subsystem1 ==
  data : Inport  OutDataTypeStr=data_type
  wr_addr : Inport  Port=2
  wr_en : Inport  Port=3
  rd_addr : Inport  Port=4
  Demux : Demux  Outputs=2
  Mux : Mux  Inputs=2
  Simple Dual Port RAM : hdlsllib/HDL RAMs/Simple Dual Port RAM  ram_size=address_len
  Simple Dual Port RAM1 : hdlsllib/HDL RAMs/Simple Dual Port RAM  ram_size=address_len
  rd_dout : Outport  PortDimensions=2  VectorParamsAs1DForOutWhenUnconnected=off
  wires:
  rd_addr/1 -> Simple Dual Port RAM1/4, Simple Dual Port RAM/4
  wr_en/1 -> Simple Dual Port RAM1/3, Simple Dual Port RAM/3
  wr_addr/1 -> Simple Dual Port RAM/2, Simple Dual Port RAM1/2
  Demux/2 -> Simple Dual Port RAM1/1
  Demux/1 -> Simple Dual Port RAM/1
  data/1 -> Demux/1
  Simple Dual Port RAM1/1 -> Mux/2
  Simple Dual Port RAM/1 -> Mux/1
  Mux/1 -> rd_dout/1

== system rx2/process9/decoder/p-p/Subsystem2/Subsystem1/Subsystem1/Subsystem1/Subsystem4/Subsystem ==
  data : Inport  OutDataTypeStr=data_type
  wr_addr : Inport  Port=2
  wr_en : Inport  Port=3
  rd_addr : Inport  Port=4
  Demux : Demux  Outputs=2
  Mux : Mux  Inputs=2
  Simple Dual Port RAM : hdlsllib/HDL RAMs/Simple Dual Port RAM  ram_size=address_len
  Simple Dual Port RAM1 : hdlsllib/HDL RAMs/Simple Dual Port RAM  ram_size=address_len
  rd_dout : Outport  PortDimensions=2  VectorParamsAs1DForOutWhenUnconnected=off
  wires:
  Mux/1 -> rd_dout/1
  Simple Dual Port RAM/1 -> Mux/1
  Simple Dual Port RAM1/1 -> Mux/2
  data/1 -> Demux/1
  Demux/1 -> Simple Dual Port RAM/1
  Demux/2 -> Simple Dual Port RAM1/1
  wr_addr/1 -> Simple Dual Port RAM1/2, Simple Dual Port RAM/2
  wr_en/1 -> Simple Dual Port RAM/3, Simple Dual Port RAM1/3
  rd_addr/1 -> Simple Dual Port RAM/4, Simple Dual Port RAM1/4

== system rx2/process9/decoder/p-p/Subsystem2/Subsystem1/Subsystem1/Subsystem1/Subsystem4/Subsystem1 ==
  data : Inport  OutDataTypeStr=data_type
  wr_addr : Inport  Port=2
  wr_en : Inport  Port=3
  rd_addr : Inport  Port=4
  Demux : Demux  Outputs=2
  Mux : Mux  Inputs=2
  Simple Dual Port RAM : hdlsllib/HDL RAMs/Simple Dual Port RAM  ram_size=address_len
  Simple Dual Port RAM1 : hdlsllib/HDL RAMs/Simple Dual Port RAM  ram_size=address_len
  rd_dout : Outport  PortDimensions=2  VectorParamsAs1DForOutWhenUnconnected=off
  wires:
  rd_addr/1 -> Simple Dual Port RAM1/4, Simple Dual Port RAM/4
  wr_en/1 -> Simple Dual Port RAM1/3, Simple Dual Port RAM/3
  wr_addr/1 -> Simple Dual Port RAM/2, Simple Dual Port RAM1/2
  Demux/2 -> Simple Dual Port RAM1/1
  Demux/1 -> Simple Dual Port RAM/1
  data/1 -> Demux/1
  Simple Dual Port RAM1/1 -> Mux/2
  Simple Dual Port RAM/1 -> Mux/1
  Mux/1 -> rd_dout/1

== system rx2/process9/decoder/p-p/Subsystem2/Subsystem1/Subsystem2/Subsystem/Subsystem1/Subsystem ==
  data : Inport  OutDataTypeStr=data_type
  wr_addr : Inport  Port=2
  wr_en : Inport  Port=3
  rd_addr : Inport  Port=4
  Demux : Demux  Outputs=2
  Mux : Mux  Inputs=2
  Simple Dual Port RAM : hdlsllib/HDL RAMs/Simple Dual Port RAM  ram_size=address_len
  Simple Dual Port RAM1 : hdlsllib/HDL RAMs/Simple Dual Port RAM  ram_size=address_len
  rd_dout : Outport  PortDimensions=2  VectorParamsAs1DForOutWhenUnconnected=off
  wires:
  Mux/1 -> rd_dout/1
  Simple Dual Port RAM/1 -> Mux/1
  Simple Dual Port RAM1/1 -> Mux/2
  data/1 -> Demux/1
  Demux/1 -> Simple Dual Port RAM/1
  Demux/2 -> Simple Dual Port RAM1/1
  wr_addr/1 -> Simple Dual Port RAM1/2, Simple Dual Port RAM/2
  wr_en/1 -> Simple Dual Port RAM/3, Simple Dual Port RAM1/3
  rd_addr/1 -> Simple Dual Port RAM/4, Simple Dual Port RAM1/4

== system rx2/process9/decoder/p-p/Subsystem2/Subsystem1/Subsystem2/Subsystem/Subsystem1/Subsystem1 ==
  data : Inport  OutDataTypeStr=data_type
  wr_addr : Inport  Port=2
  wr_en : Inport  Port=3
  rd_addr : Inport  Port=4
  Demux : Demux  Outputs=2
  Mux : Mux  Inputs=2
  Simple Dual Port RAM : hdlsllib/HDL RAMs/Simple Dual Port RAM  ram_size=address_len
  Simple Dual Port RAM1 : hdlsllib/HDL RAMs/Simple Dual Port RAM  ram_size=address_len
  rd_dout : Outport  PortDimensions=2  VectorParamsAs1DForOutWhenUnconnected=off
  wires:
  rd_addr/1 -> Simple Dual Port RAM1/4, Simple Dual Port RAM/4
  wr_en/1 -> Simple Dual Port RAM1/3, Simple Dual Port RAM/3
  wr_addr/1 -> Simple Dual Port RAM/2, Simple Dual Port RAM1/2
  Demux/2 -> Simple Dual Port RAM1/1
  Demux/1 -> Simple Dual Port RAM/1
  data/1 -> Demux/1
  Simple Dual Port RAM1/1 -> Mux/2
  Simple Dual Port RAM/1 -> Mux/1
  Mux/1 -> rd_dout/1

== system rx2/process9/decoder/p-p/Subsystem2/Subsystem1/Subsystem2/Subsystem/Subsystem4/Subsystem ==
  data : Inport  OutDataTypeStr=data_type
  wr_addr : Inport  Port=2
  wr_en : Inport  Port=3
  rd_addr : Inport  Port=4
  Demux : Demux  Outputs=2
  Mux : Mux  Inputs=2
  Simple Dual Port RAM : hdlsllib/HDL RAMs/Simple Dual Port RAM  ram_size=address_len
  Simple Dual Port RAM1 : hdlsllib/HDL RAMs/Simple Dual Port RAM  ram_size=address_len
  rd_dout : Outport  PortDimensions=2  VectorParamsAs1DForOutWhenUnconnected=off
  wires:
  rd_addr/1 -> Simple Dual Port RAM1/4, Simple Dual Port RAM/4
  wr_en/1 -> Simple Dual Port RAM1/3, Simple Dual Port RAM/3
  wr_addr/1 -> Simple Dual Port RAM/2, Simple Dual Port RAM1/2
  Demux/2 -> Simple Dual Port RAM1/1
  Demux/1 -> Simple Dual Port RAM/1
  data/1 -> Demux/1
  Simple Dual Port RAM1/1 -> Mux/2
  Simple Dual Port RAM/1 -> Mux/1
  Mux/1 -> rd_dout/1

== system rx2/process9/decoder/p-p/Subsystem2/Subsystem1/Subsystem2/Subsystem/Subsystem4/Subsystem1 ==
  data : Inport  OutDataTypeStr=data_type
  wr_addr : Inport  Port=2
  wr_en : Inport  Port=3
  rd_addr : Inport  Port=4
  Demux : Demux  Outputs=2
  Mux : Mux  Inputs=2
  Simple Dual Port RAM : hdlsllib/HDL RAMs/Simple Dual Port RAM  ram_size=address_len
  Simple Dual Port RAM1 : hdlsllib/HDL RAMs/Simple Dual Port RAM  ram_size=address_len
  rd_dout : Outport  PortDimensions=2  VectorParamsAs1DForOutWhenUnconnected=off
  wires:
  Mux/1 -> rd_dout/1
  Simple Dual Port RAM/1 -> Mux/1
  Simple Dual Port RAM1/1 -> Mux/2
  data/1 -> Demux/1
  Demux/1 -> Simple Dual Port RAM/1
  Demux/2 -> Simple Dual Port RAM1/1
  wr_addr/1 -> Simple Dual Port RAM1/2, Simple Dual Port RAM/2
  wr_en/1 -> Simple Dual Port RAM/3, Simple Dual Port RAM1/3
  rd_addr/1 -> Simple Dual Port RAM/4, Simple Dual Port RAM1/4

== system rx2/process9/decoder/p-p/Subsystem2/Subsystem1/Subsystem2/Subsystem1/Subsystem1/Subsystem ==
  data : Inport  OutDataTypeStr=data_type
  wr_addr : Inport  Port=2
  wr_en : Inport  Port=3
  rd_addr : Inport  Port=4
  Demux : Demux  Outputs=2
  Mux : Mux  Inputs=2
  Simple Dual Port RAM : hdlsllib/HDL RAMs/Simple Dual Port RAM  ram_size=address_len
  Simple Dual Port RAM1 : hdlsllib/HDL RAMs/Simple Dual Port RAM  ram_size=address_len
  rd_dout : Outport  PortDimensions=2  VectorParamsAs1DForOutWhenUnconnected=off
  wires:
  Mux/1 -> rd_dout/1
  Simple Dual Port RAM/1 -> Mux/1
  Simple Dual Port RAM1/1 -> Mux/2
  data/1 -> Demux/1
  Demux/1 -> Simple Dual Port RAM/1
  Demux/2 -> Simple Dual Port RAM1/1
  wr_addr/1 -> Simple Dual Port RAM1/2, Simple Dual Port RAM/2
  wr_en/1 -> Simple Dual Port RAM/3, Simple Dual Port RAM1/3
  rd_addr/1 -> Simple Dual Port RAM/4, Simple Dual Port RAM1/4

== system rx2/process9/decoder/p-p/Subsystem2/Subsystem1/Subsystem2/Subsystem1/Subsystem1/Subsystem1 ==
  data : Inport  OutDataTypeStr=data_type
  wr_addr : Inport  Port=2
  wr_en : Inport  Port=3
  rd_addr : Inport  Port=4
  Demux : Demux  Outputs=2
  Mux : Mux  Inputs=2
  Simple Dual Port RAM : hdlsllib/HDL RAMs/Simple Dual Port RAM  ram_size=address_len
  Simple Dual Port RAM1 : hdlsllib/HDL RAMs/Simple Dual Port RAM  ram_size=address_len
  rd_dout : Outport  PortDimensions=2  VectorParamsAs1DForOutWhenUnconnected=off
  wires:
  rd_addr/1 -> Simple Dual Port RAM1/4, Simple Dual Port RAM/4
  wr_en/1 -> Simple Dual Port RAM1/3, Simple Dual Port RAM/3
  wr_addr/1 -> Simple Dual Port RAM/2, Simple Dual Port RAM1/2
  Demux/2 -> Simple Dual Port RAM1/1
  Demux/1 -> Simple Dual Port RAM/1
  data/1 -> Demux/1
  Simple Dual Port RAM1/1 -> Mux/2
  Simple Dual Port RAM/1 -> Mux/1
  Mux/1 -> rd_dout/1

== system rx2/process9/decoder/p-p/Subsystem2/Subsystem1/Subsystem2/Subsystem1/Subsystem4/Subsystem ==
  data : Inport  OutDataTypeStr=data_type
  wr_addr : Inport  Port=2
  wr_en : Inport  Port=3
  rd_addr : Inport  Port=4
  Demux : Demux  Outputs=2
  Mux : Mux  Inputs=2
  Simple Dual Port RAM : hdlsllib/HDL RAMs/Simple Dual Port RAM  ram_size=address_len
  Simple Dual Port RAM1 : hdlsllib/HDL RAMs/Simple Dual Port RAM  ram_size=address_len
  rd_dout : Outport  PortDimensions=2  VectorParamsAs1DForOutWhenUnconnected=off
  wires:
  Mux/1 -> rd_dout/1
  Simple Dual Port RAM/1 -> Mux/1
  Simple Dual Port RAM1/1 -> Mux/2
  data/1 -> Demux/1
  Demux/1 -> Simple Dual Port RAM/1
  Demux/2 -> Simple Dual Port RAM1/1
  wr_addr/1 -> Simple Dual Port RAM1/2, Simple Dual Port RAM/2
  wr_en/1 -> Simple Dual Port RAM/3, Simple Dual Port RAM1/3
  rd_addr/1 -> Simple Dual Port RAM/4, Simple Dual Port RAM1/4

== system rx2/process9/decoder/p-p/Subsystem2/Subsystem1/Subsystem2/Subsystem1/Subsystem4/Subsystem1 ==
  data : Inport  OutDataTypeStr=data_type
  wr_addr : Inport  Port=2
  wr_en : Inport  Port=3
  rd_addr : Inport  Port=4
  Demux : Demux  Outputs=2
  Mux : Mux  Inputs=2
  Simple Dual Port RAM : hdlsllib/HDL RAMs/Simple Dual Port RAM  ram_size=address_len
  Simple Dual Port RAM1 : hdlsllib/HDL RAMs/Simple Dual Port RAM  ram_size=address_len
  rd_dout : Outport  PortDimensions=2  VectorParamsAs1DForOutWhenUnconnected=off
  wires:
  rd_addr/1 -> Simple Dual Port RAM1/4, Simple Dual Port RAM/4
  wr_en/1 -> Simple Dual Port RAM1/3, Simple Dual Port RAM/3
  wr_addr/1 -> Simple Dual Port RAM/2, Simple Dual Port RAM1/2
  Demux/2 -> Simple Dual Port RAM1/1
  Demux/1 -> Simple Dual Port RAM/1
  data/1 -> Demux/1
  Simple Dual Port RAM1/1 -> Mux/2
  Simple Dual Port RAM/1 -> Mux/1
  Mux/1 -> rd_dout/1
